simulink library "func_lib"  (R2024b)
settings: Solver=VariableStepAuto  StartTime=0.0  StopTime=10.0  RelTol=1e-3
settings Model: Creator=shunx  LastModifiedBy=shunx

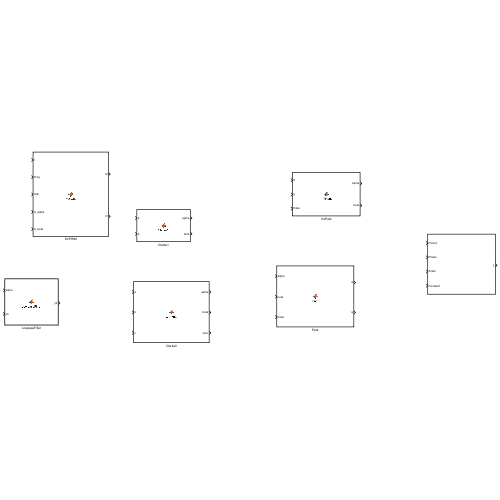
[thumbnail: Simulink's stored preview of the top-level diagram]
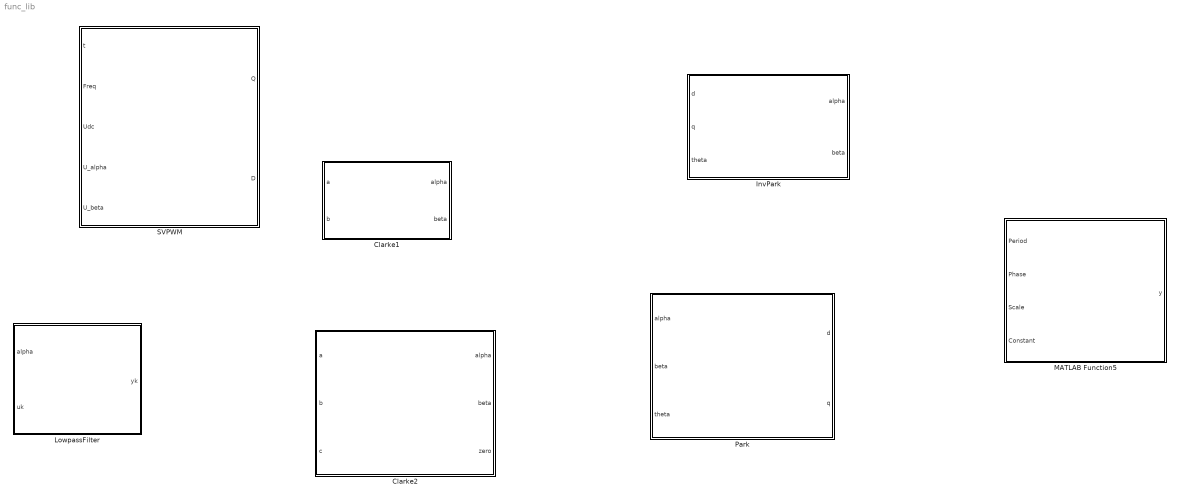
== system func_lib ==
  Clarke1 : MATLAB Function  TreatAsAtomicUnit=on
  Clarke2 : MATLAB Function  TreatAsAtomicUnit=on
  InvPark : MATLAB Function  TreatAsAtomicUnit=on
  LowpassFilter : MATLAB Function  TreatAsAtomicUnit=on
  MATLAB Function5 : MATLAB Function  TreatAsAtomicUnit=on
  Park : MATLAB Function  TreatAsAtomicUnit=on
  SVPWM : MATLAB Function  TreatAsAtomicUnit=on

== matlab function func_lib/Clarke1 ==
  data: a input; alpha output; b input; beta output
function [alpha, beta] = Clarke1(a, b)
alpha= a;
beta= a/sqrt(3) + 2 * b / sqrt(3);

== matlab function func_lib/SVPWM ==
  data: t input; Freq input; Q output; Udc input; U_alpha input; U_beta input; D output
% 仿真时间
% Freq: pwm频率
% Udc: 母线电压
% U_alpha: alpha轴电压
% U_beta: beta轴电压
% Q: 6路pwm开关输出 [Q1 /Q1 Q2 /Q2 Q3 /Q3]
% D: ABC相上桥臂PWM占空比
function [Q, D] = svpwm(t, Freq, Udc, U_alpha, U_beta)
    persistent svpwmSectorTab;
    persistent pwmCompareTab;
	persistent pwmPeriad;
    persistent ABC;
    persistent T12;
    persistent Tabc;
    persistent CompareABCIndex;
	persistent LastUpdateTime;

	if isempty(pwmCompareTab)
		pwmCompareTab = [1 2 3;2 1 3;3 1 2;3 2 1;2 3 1;1 3 2]';
	end
	if isempty(svpwmSectorTab)
		svpwmSectorTab = [2 6 1 4 3 5];
	end
	if isempty(pwmPeriad)
		pwmPeriad = 1/Freq;
	end
	if isempty(Tabc)
		Tabc = [0 0 0]';
	end
	if isempty(T12)
		T12 = [0 0]';
	end
	if isempty(ABC)
		ABC = [0 0 0]';
	end
	if isempty(CompareABCIndex)
		CompareABCIndex = [0 0 0]';
	end
	if isempty(LastUpdateTime)
		LastUpdateTime =  -pwmPeriad;
	end

    % 每个PWM周期才计算一次
	% 并更新LastUpdateTime
    if (t - LastUpdateTime) >= pwmPeriad
		LastUpdateTime = t;
        % 计算A，B，C
        ABC = [0 1; sqrt(3)/2 -1/2; -sqrt(3)/2 -1/2] * [U_alpha, U_beta]';
        XYZ = zeros(3,1);
        for i = 1:3
            if ABC(i,1) > 0
                XYZ(i,1) = 1;
            else
                XYZ(i, 1) = 0;
            end
        end
        N = 4 * XYZ(3,1) + 2 * XYZ(2,1) + XYZ(1,1);
		if N == 0
			N = 1;
		end
		% 更新 CompareABCIndex, pwmSectorTab(N)即为扇区号
		CompareABCIndex = pwmCompareTab(:, svpwmSectorTab(N));
		% 更新 T12
        switch svpwmSectorTab(N)
            case 1
                T12 = 2*pwmPeriad/sqrt(3) / Udc * [ABC(2) ABC(1)]';
            case 2
                T12 = 2*pwmPeriad/sqrt(3) / Udc * [-ABC(2) -ABC(3)]';
            case 3
                T12 = 2*pwmPeriad/sqrt(3) / Udc * [ABC(1) ABC(3)]';
            case 4
                T12 = 2*pwmPeriad/sqrt(3) / Udc * [-ABC(1) -ABC(2)]';
            case 5
                T12 = 2*pwmPeriad/sqrt(3) / Udc * [ABC(3) ABC(2)]';
            case 6
                T12 = 2*pwmPeriad/sqrt(3) / Udc * [-ABC(3) -ABC(1)]';
        end
		if sum(T12) > pwmPeriad
			T12 = pwmPeriad * T12 / sum(T12);
		end
		%更新Tabc
        Tabc = [-1/4 -1/4;1/4 -1/4; 1/4 1/4] * T12 + [pwmPeriad/4 pwmPeriad/4 pwmPeriad/4]';
    end
    
    Q = zeros(6,1);
	D = zeros(3,1);
	D(:,1) = Tabc(CompareABCIndex(:, 1), 1);

    for i = 1:3
        if (t - LastUpdateTime) > D(i,1) && (t - LastUpdateTime) <= (pwmPeriad - D(i,1))
            Q((i-1)*2+1,1) = 1;
            Q((i-1)*2+2,1) = 0;
		else 
            Q((i-1)*2+1,1) = 0;
            Q((i-1)*2+2,1) = 1;
        end
    end

== matlab function func_lib/Clarke2 ==
  data: a input; alpha output; b input; c input; beta output; zero output
function [alpha, beta, zero ] = Clarke2(a, b, c)
alpha = (a - 0.5*b - 0.5*c) * 2 /3;
beta = 2/3 * ( sqrt(3) * 0.5 * b - sqrt(3)*0.5*c );
zero = 2/3 * (0.5*a + 0.5*b + 0.5*c);

== matlab function func_lib/Park ==
  data: alpha input; d output; beta input; theta input; q output
function [d, q] = Park(alpha, beta, theta)
d = cos(theta)* alpha + sin(theta) * beta;
q = -sin(theta)* alpha + cos(theta) * beta;

== matlab function func_lib/InvPark ==
  data: d input; alpha output; q input; theta input; beta output
function [alpha, beta] = InvPark(d, q, theta)
alpha = d*cos(theta) - q*sin(theta);
beta  = d*sin(theta) + q*cos(theta);

== matlab function func_lib/MATLAB Function5 ==
  data: Period input; y output; Phase input; Scale input; Constant input
function y = TriangleWave(Period, Phase, Scale, Constant)
    % 声明外部函数以获取仿真时间
    coder.extrinsic('get_param');
    simtime = 0;  % 初始化仿真时间变量
    simtime = get_param(bdroot, 'SimulationTime');  % 获取当前仿真时间

    persistent kline;
    persistent TimeOfPhase;
    if isempty(kline)
        kline = 4*Scale/Period;
    end
    if isempty(TimeOfPhase)
        TimeOfPhase = Period * Phase*0.5/pi;
    end

    simtime = simtime + TimeOfPhase;
    
    if mod(simtime, Period) < (Period*0.5)
        y = -Scale + kline * mod(simtime, Period);
    else
        y = Scale - kline * (mod(simtime, Period) - Period*0.5);
    end

    y = y + Constant;

== matlab function func_lib/LowpassFilter ==
  data: alpha input; yk output; uk input
function yk = LowpassFilter(alpha, uk)
persistent preUk;

if isempty(preUk)
	preUk = 0;
end

yk = alpha * uk + (1-alpha) * preUk;
